simulink library "spoolOutSpoolingController_ul"  (R2020a)
settings: Solver=VariableStepAuto  StartTime=0.0  StopTime=10.0  RelTol=1e-3
undefined symbols (not defined in the file or in its folder): pathCtrl
settings Model: Creator=James Reed  LastModifiedBy=Josh Gaming
settings DataIOCC: ReturnWorkspaceOutputs=off
settings DebuggingCC: ArithmeticOperatorsInVariantConditions=warning
settings SFSimCC: CustomCodeUndefinedFunction=UseInterfaceOnly

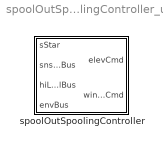
== system spoolOutSpoolingController_ul ==
  spoolOutSpoolingController : Subsystem

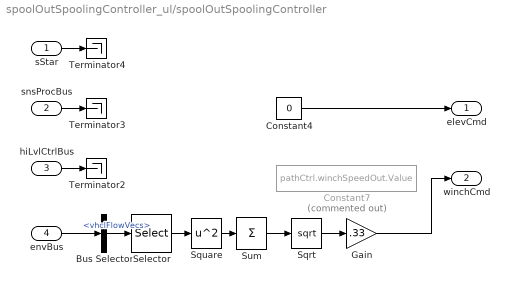
== system spoolOutSpoolingController_ul/spoolOutSpoolingController ==
  "sStar " : Inport
  snsProcBus : Inport  Port=2  OutDataTypeStr=Bus: sensorsProcessingBus
  hiLvlCtrlBus : Inport  Port=3  OutDataTypeStr=Bus: hiLvlCtrlBus
  envBus : Inport  Port=4  OutDataTypeStr=Bus: envBus
  Bus Selector : BusSelector  OutputSignals=vhclFlowVecs
  Constant4 : Constant  Value=0
  Constant7 : Constant  Commented=on  Value=pathCtrl.winchSpeedOut.Value
  Gain : Gain  Gain=.33
  Selector : Selector  NumberOfDimensions=2  InputPortWidth=3  IndexOptions=Select all,Index vector (dialog)  Indices=[1 3],5  OutputSizes=1,1
  Sqrt : Sqrt  SaturateOnIntegerOverflow=on
  Square : Math  Operator=square  SaturateOnIntegerOverflow=on
  Sum : Sum  Inputs=+
  Terminator2 : Terminator
  Terminator3 : Terminator
  Terminator4 : Terminator
  elevCmd : Outport  VectorParamsAs1DForOutWhenUnconnected=off
  "winchCmd " : Outport  Port=2  VectorParamsAs1DForOutWhenUnconnected=off
  wires:
  hiLvlCtrlBus/1 -> Terminator2/1
  Constant4/1 -> elevCmd/1
  envBus/1 -> Bus Selector/1
  snsProcBus/1 -> Terminator3/1
  "sStar "/1 -> Terminator4/1
  Bus Selector/1 -> Selector/1  "<vhclFlowVecs>"
  Square/1 -> Sum/1
  Sum/1 -> Sqrt/1
  Sqrt/1 -> Gain/1
  Gain/1 -> "winchCmd "/1
  Selector/1 -> Square/1
